simulink model "sscfluids_clutch_ss_primary_cyl"  (R2021b)
settings: Solver=VariableStepAuto  StartTime=0.0  StopTime=simT  RelTol=1e-3  AbsTol=1e-3
PreLoadFcn:
  | sscfluids_clutch_ss_primary_cyl_input
undefined symbols (not defined in the file): sspc
libraries: fl_lib x12, nesl_utility x3, SimscapeFluids_lib x2, simulink x1
CloseFcn:
  | clear logsout_sscfluids_clutch_ss_primary_cyl
  | clear simT ii jj sspc tout
  | clear simlog_sscfluids_clutch_ss_primary_cyl
  | 
  | try,close(h_sscfluids_clutch_ss_primary_cyl),end
  | clear h_sscfluids_clutch_ss_primary_cyl
Description:
  | Single-Stage Primary Cylinder
settings Model: Creator=The MathWorks, Inc.  LastModifiedBy=pgzar
settings SolverCC: AutoScaleAbsTol=off  AlgebraicLoopSolver=TrustRegion
settings DataIOCC: MaxDataPoints=10000  DSMLogging=off  SaveTime=off  ReturnWorkspaceOutputs=off  OutputSaveName=logsout_sscfluids_clutch_ss_primary_cyl  SignalLoggingName=logsout_sscfluids_clutch_ss_primary_cyl
settings DebuggingCC: SymbolicDimsDataTypeCodeGenerationDiagnostic=none  SFMachineParentedDataDiag=warning
settings SFSimCC: CustomCodeUndefinedFunction=UseInterfaceOnly
settings SimscapeCC: SimscapeLogType=all  SimscapeLogSimulationStatistics=on  SimscapeLogName=simlog_sscfluids_clutch_ss_primary_cyl  SimscapeLogDataHistory=100000

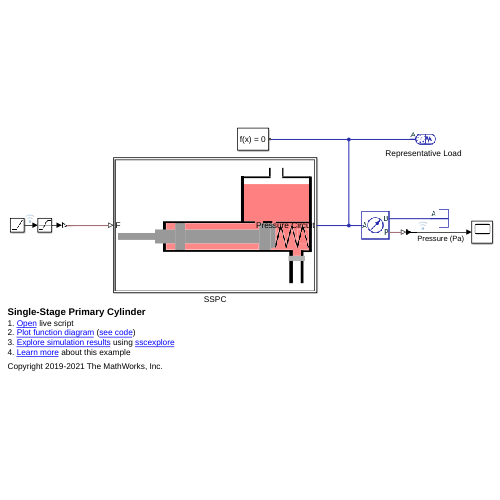
[thumbnail: Simulink's stored preview of the top-level diagram]
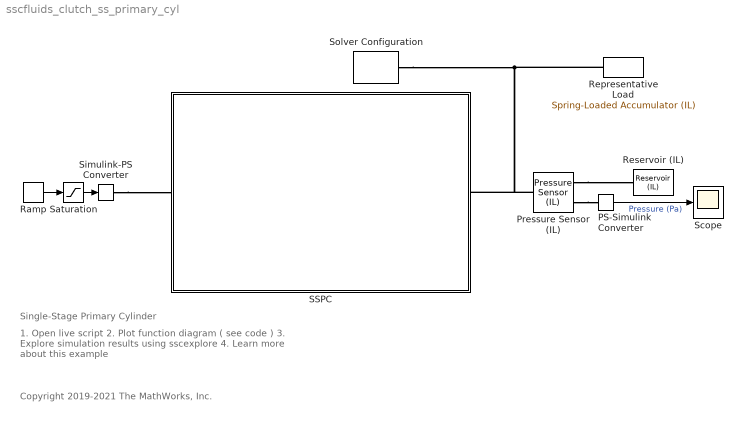
== system sscfluids_clutch_ss_primary_cyl ==
  note: Single-Stage Primary Cylinder
  note: 1. Open live script
      | 2. Plot function diagram ( see code )
      | 3. Explore simulation results using sscexplore
      | 4. Learn more about this example
  note: Copyright 2019-2021 The MathWorks, Inc.
  PS-Simulink Converter : nesl_utility/PS-Simulink Converter  PhysicalDomain=network_engine_domain  SubClassName=ps_output  LeftPortType=input  RightPortType=output  PseudoPeriodic=off  Frequencies=[]  Unit=Pa  AffineConversion=off
      settings: SourceProductBaseCode=PW,SS
  Pressure Sensor (IL) : fl_lib/Isothermal Liquid/Sensors/Pressure Sensor (IL)  pressure_measure=foundation.enum.pressure_measure.difference
      settings: SourceProductBaseCode=SS  InternalSimscapePortConfiguration="{\"Bottom\":[],\"Left\":[{\"id\":\"A\",\"label\":\"A\",\"type\":\"foundation.isothermal_liquid.isothermal_liquid\"}],\"Right\":[{\"id\":\"B\",\"label\":\"B\",\"type\":\"foundation.isothermal_liquid.isothermal_liquid\"},{\"id\":\"P\",\"label\":\"P\",\"type\":\"output\"}],\"Top\":[]}"
  Ramp : simulink/Sources/Ramp  slope=25  start=1  InitialOutput=0
  Representative Load : SimscapeFluids_lib/Isothermal Liquid/Tanks & Accumulators/Spring-Loaded Accumulator (IL)  capacity=sspc.vol m^3  p_preload=sspc.pRes Pa  p_max=sspc.loadP Pa  stiff_coeff=1e10 Pa/m^3  dynamic_compressibility=simscape.enum.onoff.on  liquid_volume_specify=off  liquid_volume_priority=High  liquid_volume=0.005 m^3  liquid_volume_nominal_specify=off  liquid_volume_nominal_unit=m^3  liquid_volume_nominal_value=1  liquid_mass_specify=off  liquid_mass_priority=None  liquid_mass=5 kg  liquid_mass_nominal_specify=off  liquid_mass_nominal_unit=kg  liquid_mass_nominal_value=1  p_I_specify=off  p_I_priority=None  p_I=0.101325 MPa  p_I_nominal_specify=off  p_I_nominal_unit=MPa  p_I_nominal_value=1
      settings: SourceProductBaseCode=SH  InternalSimscapePortConfiguration="{\"Bottom\":[],\"Left\":[],\"Right\":[{\"id\":\"A\",\"label\":\"A\",\"type\":\"foundation.isothermal_liquid.isothermal_liquid\"}],\"Top\":[]}"
  Reservoir (IL) : fl_lib/Isothermal Liquid/Elements/Reservoir (IL)  reservoir_type=foundation.enum.constant_controlled.constant  pressure_spec=foundation.enum.pressure_spec.atmospheric  reservoir_pressure=0.101325 MPa
      settings: SourceProductBaseCode=SS
  SSPC : Subsystem
      mask Display:
      | port_label('RConn',1,'Pressure')
      | port_label('LConn',1,'PRF')
      | image('sscfluids_clutch_ss_primary_cyl.png');
  Saturation : Saturate  UpperLimit=sspc.pushRodF(3)  LowerLimit=0
  Scope : Scope
  Simulink-PS Converter : nesl_utility/Simulink-PS Converter  PhysicalDomain=network_engine_domain  SubClassName=ps_input  LeftPortType=input  RightPortType=output  PseudoPeriodic=off  Frequencies=[]  NoiseDistribution=none  NoiseParameters=[]  Unit=N  AffineConversion=off  FilteringAndDerivatives=provide  SimscapeFilterOrder=1  InputFilterTimeConstant=0.001  UdotUserProvided=0
      settings: SourceProductBaseCode=PW,SS
  Solver Configuration : nesl_utility/Solver Configuration  PhysicalDomain=network_engine_domain  SubClassName=solver  LeftPortType=input  RightPortType=generic  Tones=[]  Harmonics=[]  SimulateNoise=off  Profile=off  UseLocalSampling=off  EnableSwitchedLinearOptims=on  FrequencyDomain=off  UseCCode=off  RelTol=0.001  AbsTol=1e-06  MinStep=1e-09  ToWorkspace=off  RevertToSquareIcSolve=off  NumHomotopyIterations=100  PhasorMode=off  PhasorModeNumHarmonics=1  DoDC=on  ResidualTolerance=1e-9  UseLocalSolver=off  LocalSolverChoice=NE_BACKWARD_EULER_ADVANCER  LocalSolverSampleTime=0.001  DoFixedCost=off  MaxNonlinIter=3  MaxModeIter=2  ComputeImpulses=off  ImpulseIterations=2  LinearAlgebra=auto  EquationFormulation=NE_TIME_EF  DelaysMemoryBudget=1024  AutomaticFiltering=on  FilteringTimeConstant=0.001  PartitionStorageMethod=AS_NEEDED  PartitionMemoryBudget=1024  PartitionMethod=FAST
      settings: SourceProductBaseCode=PW,SS
  wires:
  Saturation/1 -> Simulink-PS Converter/1
  Ramp/1 -> Saturation/1
  PS-Simulink Converter/1 -> Scope/1  "Pressure (Pa)"
  connections:
  Solver Configuration/RConn1 -- Representative Load/RConn1 -- SSPC/RConn1 -- Pressure Sensor (IL)/LConn1
  Simulink-PS Converter/RConn1 -- SSPC/LConn1
  Pressure Sensor (IL)/RConn1 -- Reservoir (IL)/LConn1
  Pressure Sensor (IL)/RConn2 -- PS-Simulink Converter/LConn1

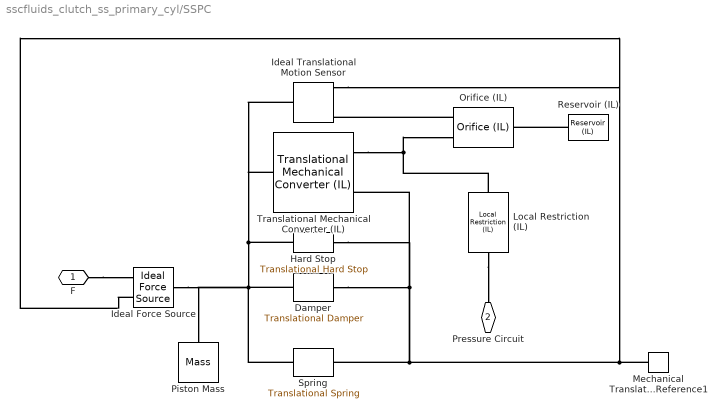
== system sscfluids_clutch_ss_primary_cyl/SSPC ==
  Damper : fl_lib/Mechanical/Translational Elements/Translational Damper  D=sspc.c N/(m/s)  v_specify=off  v_priority=None  v=0 m/s  v_nominal_specify=off  v_nominal_unit=m/s  v_nominal_value=1  f_specify=off  f_priority=None  f=0 N  f_nominal_specify=off  f_nominal_unit=N  f_nominal_value=1
  Hard Stop : fl_lib/Mechanical/Translational Elements/Translational Hard Stop  upper_bnd=sspc.stroke m  lower_bnd=0 m  stiff_up=sspc.hss N/m  stiff_low=sspc.hss N/m  D_up=sspc.hsd N/(m/s)  D_low=sspc.hsd N/(m/s)  model=simscape.enum.hardstop.smooth  transition=0.1 mm  v_specify=off  v_priority=None  v=0 m/s  v_nominal_specify=off  v_nominal_unit=m/s  v_nominal_value=1  f_specify=off  f_priority=None  f=0 N  f_nominal_specify=off  f_nominal_unit=N  f_nominal_value=1  x_specify=off  x_priority=High  x=0 m  x_nominal_specify=off  x_nominal_unit=m  x_nominal_value=1
  Ideal Force Source : fl_lib/Mechanical/Mechanical Sources/Ideal Force Source
  Ideal Translational Motion Sensor : fl_lib/Mechanical/Mechanical Sensors/Ideal Translational Motion Sensor  offset=0 m
  Local Restriction (IL) : fl_lib/Isothermal Liquid/Elements/Local Restriction (IL)  restriction_type=foundation.enum.restriction_type.fixed  restriction_area=sspc.a2Ori m^2  min_area=1e-10 m^2  max_area=0.005 m^2  area=inf m^2  Cd=0.7  Re_c=12  pressure_recovery=simscape.enum.onoff.off
      settings: SourceProductBaseCode=SS  InternalSimscapePortConfiguration="{\"Bottom\":[],\"Left\":[{\"id\":\"A\",\"label\":\"A\",\"type\":\"foundation.isothermal_liquid.isothermal_liquid\"}],\"Right\":[{\"id\":\"B\",\"label\":\"B\",\"type\":\"foundation.isothermal_liquid.isothermal_liquid\"}],\"Top\":[]}"
  Mechanical Translational Reference1 : fl_lib/Mechanical/Translational Elements/Mechanical Translational Reference
  Orifice (IL) : SimscapeFluids_lib/Isothermal Liquid/Valves & Orifices/Orifices/Orifice (IL)  orifice_type=foundation.enum.constant_variable.variable  constant_orifice_spec=fluids.isothermal_liquid.valves_orifices.orifices.enum.constant_orifice_spec.area  variable_orifice_spec=fluids.isothermal_liquid.valves_orifices.orifices.enum.orifice_spec.table1D_area_opening  orifice_area_constant=1e-3 m^2  p_diff_TLU_constant=[-4, -3, -2, -1, -.5, 0, .5, 1, 2, 3, 4] MPa  vol_flow_TLU_constant=[-2.44, -2.12, -1.68, -1.22, -.84, 0, .85, 1.21, 1.7, 2.09, 2.41] .* 1e-3 m^3/s  S_min=0 m  del_S=5e-3 m  open_orientation=fluids.isothermal_liquid.valves_orifices.orifices.enum.orifice_orientation.positive  area_max=1e-4 m^2  area_leak=1e-10 m^2  S_TLU=[0 sspc.deadzone sspc.stroke] m  orifice_area_TLU=[sspc.a1Ori 1e-10 1e-10] m^2  area=inf m^2  Cd=0.7  Re_c=12  smoothing_factor=0.01  pressure_recovery=simscape.enum.onoff.off  S_vol_flow_TLU=[0, .002, .004, .007, .017] m  p_diff_TLU=[.3, .5, .7] MPa  vol_flow_TLU=1e-3 * [1.7e-05, 2e-05, 2.6e-05; .0035, .0045, .0053; .7, .9, 1.06; 1.96, 2.5, 3; 6, 7.7, 9.13] m^3/s  enable_faults=simscape.enum.onoff.off  fault_action=fluids.enum.FaultOpening.Closed  external_fault=fluids.enum.FaultExternalTrigger.Off  temporal_fault=simscape.enum.onoff.off  fault_time=5 s  report_fault=simscape.enum.assert.action.none  mdot_A_specify=off  mdot_A_priority=None  mdot_A=0 kg/s  mdot_A_nominal_specify=off  mdot_A_nominal_unit=kg/s  mdot_A_nominal_value=1  mdot_B_specify=off  mdot_B_priority=None  mdot_B=0 kg/s  mdot_B_nominal_specify=off  mdot_B_nominal_unit=kg/s  mdot_B_nominal_value=1
      settings: SourceProductBaseCode=SH  InternalSimscapePortConfiguration="{\"Bottom\":[],\"Left\":[{\"id\":\"A\",\"label\":\"A\",\"type\":\"foundation.isothermal_liquid.isothermal_liquid\"},{\"id\":\"S\",\"label\":\"S\",\"type\":\"input\"}],\"Right\":[{\"id\":\"B\",\"label\":\"B\",\"type\":\"foundation.isothermal_liquid.isothermal_liquid\"}],\"Top\":[]}"
  Piston Mass : fl_lib/Mechanical/Translational Elements/Mass  mass=sspc.mass kg  num_ports=foundation.enum.numPorts2.one  v_specify=off  v_priority=High  v=0 m/s  v_nominal_specify=off  v_nominal_unit=m/s  v_nominal_value=1  f_specify=off  f_priority=None  f=0 N  f_nominal_specify=off  f_nominal_unit=N  f_nominal_value=1
  Reservoir (IL) : fl_lib/Isothermal Liquid/Elements/Reservoir (IL)  reservoir_type=foundation.enum.constant_controlled.constant  pressure_spec=foundation.enum.pressure_spec.atmospheric  reservoir_pressure=0.101325 MPa
      settings: SourceProductBaseCode=SS
  Spring : fl_lib/Mechanical/Translational Elements/Translational Spring  spr_rate=sspc.k N/m  v_specify=off  v_priority=None  v=0 m/s  v_nominal_specify=off  v_nominal_unit=m/s  v_nominal_value=1  f_specify=off  f_priority=None  f=0 N  f_nominal_specify=off  f_nominal_unit=N  f_nominal_value=1  x_specify=on  x_priority=High  x=sspc.def m  x_nominal_specify=off  x_nominal_unit=m  x_nominal_value=1
  Translational Mechanical Converter (IL) : fl_lib/Isothermal Liquid/Elements/Translational Mechanical Converter (IL)  mech_orientation=foundation.enum.MechOrientationTranslational.Negative  displacement_spec=foundation.enum.DisplacementSpec.Calculate  x0=-sspc.stroke m  interface_area=sspc.aPist m^2  dead_volume=sspc.v2D m^3  pressure_spec=foundation.enum.pressure_spec.atmospheric  environment_pressure=0.101325 MPa  dynamic_compressibility=simscape.enum.onoff.on  p0=sspc.pRes Pa
      settings: SourceProductBaseCode=SS  InternalSimscapePortConfiguration="{\"Bottom\":[],\"Left\":[{\"id\":\"A\",\"label\":\"A\",\"type\":\"foundation.isothermal_liquid.isothermal_liquid\"},{\"id\":\"C\",\"label\":\"C\",\"type\":\"foundation.mechanical.translational.translational\"}],\"Right\":[{\"id\":\"R\",\"label\":\"R\",\"type\":\"foundation.mechanical.translational.translational\"}],\"Top\":[]}"
  F : PMIOPort  Side=Left
  Pressure Circuit : PMIOPort  Port=2  Side=Right
  connections:
  F/RConn1 -- Ideal Force Source/RConn1
  Damper/RConn1 -- Ideal Force Source/RConn2 -- Ideal Translational Motion Sensor/RConn1 -- Mechanical Translational Reference1/LConn1 -- Spring/RConn1 -- Translational Mechanical Converter (IL)/LConn2 -- Hard Stop/RConn1
  Spring/LConn1 -- Hard Stop/LConn1 -- Translational Mechanical Converter (IL)/RConn1 -- Ideal Translational Motion Sensor/LConn1 -- Piston Mass/LConn1 -- Ideal Force Source/LConn1 -- Damper/LConn1
  Orifice (IL)/LConn2 -- Ideal Translational Motion Sensor/RConn3
  Local Restriction (IL)/RConn1 -- Pressure Circuit/RConn1
  Translational Mechanical Converter (IL)/LConn1 -- Local Restriction (IL)/LConn1 -- Orifice (IL)/LConn1
  Reservoir (IL)/LConn1 -- Orifice (IL)/RConn1
